simulink model "c172p"  (R2026a)
settings: configuration reference "standardSILConfiguraitonParams" (kept outside this file)
undefined symbols (not defined in the file): actuatorDelay_s, plantSampleTime_s
settings Model: Creator=GTAR  LastModifiedBy=Edison Altamirano
settings ConfigSetRef: SourceName=standardSILConfiguraitonParams  SourceLocation=Base Workspace

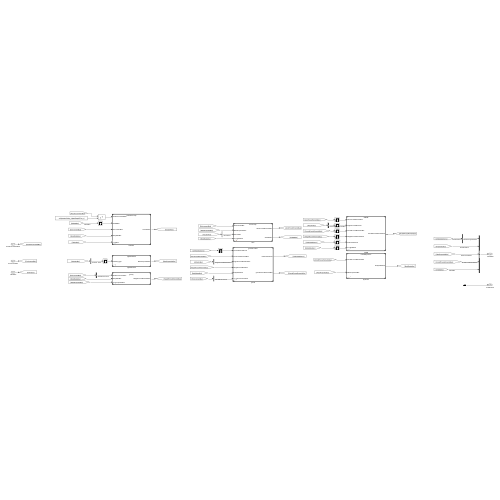
[thumbnail: Simulink's stored preview of the top-level diagram]
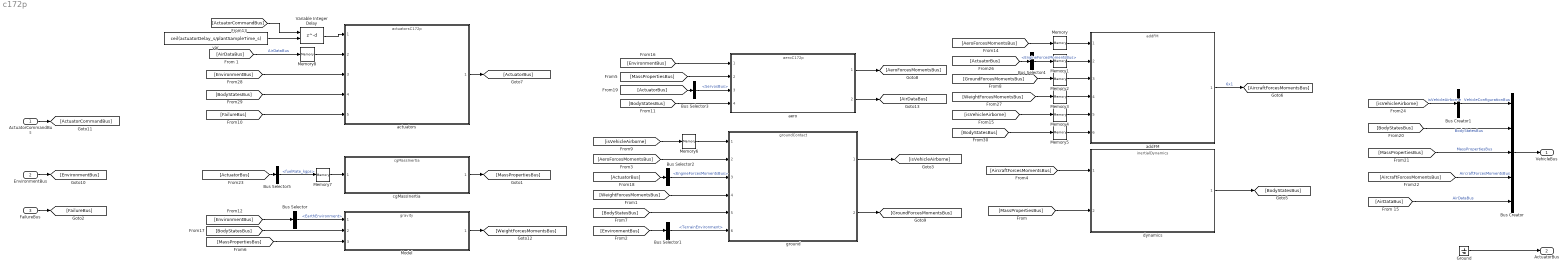
== system c172p ==
  ActuatorCommandBus : Inport  OutDataTypeStr=Bus: ActuatorCommandBus
  EnvironmentBus : Inport  Port=2  OutDataTypeStr=Bus: EnvironmentBus
  FailureBus : Inport  Port=3  OutDataTypeStr=Bus: FailureBus
  Bus Creator : BusCreator  Inputs=5  OutDataTypeStr=Bus: VehicleBus
  Bus Creator1 : BusCreator  Inputs=1  OutDataTypeStr=Bus: VehicleConfigurationBus
      settings: InheritFromInputs=off
  Bus Selector : BusSelector  OutputSignals=EarthEnvironment
  Bus Selector1 : BusSelector  OutputSignals=TerrainEnvironment
  Bus Selector2 : BusSelector  OutputSignals=PropulsionBus.EngineForcesMomentsBus
  Bus Selector3 : BusSelector  OutputSignals=ServosBus
  Bus Selector4 : BusSelector  OutputSignals=PropulsionBus.EngineForcesMomentsBus
  Bus Selector5 : BusSelector  OutputSignals=PropulsionBus.fuelRate_kgps
  Ground : Ground
  Memory{,1..8} (9 alike) : Memory
  Model : ModelReference  ModelNameDialog=gravity.slx  SimulationMode=Normal  ModelReferenceVersion=1.28
  Variable Integer Delay : Delay  DelayLengthSource=Input port
      settings: InputPortMap=u0,p1
  actuators : ModelReference  ModelNameDialog=actuatorsC172p.slx  SimulationMode=Normal  ModelReferenceVersion=5.0
  addFM : ModelReference  ModelNameDialog=addFM.slx  SimulationMode=Normal  ModelReferenceVersion=1.82
  aero : ModelReference  ModelNameDialog=aeroC172p.slx  SimulationMode=Normal  ModelReferenceVersion=5.0
  cgMassInertia : ModelReference  ModelNameDialog=cgMassInertia.slx  SimulationMode=Normal  ModelReferenceVersion=1.43
  dynamics : ModelReference  ModelNameDialog=inertialDynamics.slx  SimulationMode=Normal  ModelReferenceVersion=1.35
  ground : ModelReference  ModelNameDialog=groundContact.slx  SimulationMode=Normal  ModelReferenceVersion=1.99
  var : Constant  Value=ceil(actuatorDelay_s/plantSampleTime_s)
  VehicleBus : Outport  OutDataTypeStr=Bus: VehicleBus
  ActuatorBus : Outport  Port=2  OutDataTypeStr=Bus: ActuatorBus
  wires:
  actuators/1 -> [ActuatorBus]
  var/1 -> Variable Integer Delay/2
  Bus Selector3/1 -> aero/3  "<ServosBus>"
  [MassPropertiesBus] -> dynamics/2
  [MassPropertiesBus] -> aero/2
  Bus Creator/1 -> VehicleBus/1
  Variable Integer Delay/1 -> actuators/1
  addFM/1 -> [AircraftForcesMomentsBus]  "6x1"
  aero/1 -> [AeroForcesMomentsBus]
  [BodyStatesBus] -> aero/4
  EnvironmentBus/1 -> [EnvironmentBus]
  ActuatorCommandBus/1 -> [ActuatorCommandBus]
  [ActuatorCommandBus] -> Variable Integer Delay/1
  [AeroForcesMomentsBus] -> Memory/1
  [EnvironmentBus] -> aero/1
  Model/1 -> [WeightForcesMomentsBus]
  Bus Selector4/1 -> Memory1/1  "<EngineForcesMomentsBus>"
  [GroundForcesMomentsBus] -> Memory2/1
  ground/2 -> [GroundForcesMomentsBus]
  cgMassInertia/1 -> [MassPropertiesBus]
  ground/1 -> [isVehicleAirborne]
  Memory6/1 -> ground/1
  [isVehicleAirborne] -> Memory6/1
  [MassPropertiesBus] -> Model/3
  [EnvironmentBus] -> Bus Selector/1
  Bus Selector/1 -> Model/1  "<EarthEnvironment>"
  [BodyStatesBus] -> Model/2
  [EnvironmentBus] -> Bus Selector1/1
  [ActuatorBus] -> Bus Selector2/1
  [ActuatorBus] -> Bus Selector3/1
  [BodyStatesBus] -> Bus Creator/2  "BodyStatesBus"
  [MassPropertiesBus] -> Bus Creator/3  "MassPropertiesBus"
  [AircraftForcesMomentsBus] -> Bus Creator/4  "AircraftForcesMomentsBus"
  Bus Creator1/1 -> Bus Creator/1  "VehicleConfigurationBus"
  [isVehicleAirborne] -> Bus Creator1/1  "isVehicleAirborne"
  [ActuatorBus] -> Bus Selector4/1
  dynamics/1 -> [BodyStatesBus]
  aero/2 -> [AirDataBus]
  [AirDataBus] -> Bus Creator/5  "AirDataBus"
  [AircraftForcesMomentsBus] -> dynamics/1
  [ActuatorBus] -> Bus Selector5/1
  Bus Selector5/1 -> Memory7/1  "<fuelRate_kgps>"
  Memory7/1 -> cgMassInertia/1
  [WeightForcesMomentsBus] -> Memory3/1
  [AirDataBus] -> Memory8/1  "AirDataBus"
  [EnvironmentBus] -> actuators/3
  [BodyStatesBus] -> actuators/4
  Memory8/1 -> actuators/2
  [isVehicleAirborne] -> Memory4/1
  [BodyStatesBus] -> Memory5/1
  Ground/1 -> ActuatorBus/1
  [AeroForcesMomentsBus] -> ground/2
  Bus Selector2/1 -> ground/3  "<EngineForcesMomentsBus>"
  [WeightForcesMomentsBus] -> ground/4
  [BodyStatesBus] -> ground/5
  Bus Selector1/1 -> ground/6  "<TerrainEnvironment>"
  FailureBus/1 -> [FailureBus]
  [FailureBus] -> actuators/5
  Memory2/1 -> addFM/3
  Memory/1 -> addFM/1
  Memory1/1 -> addFM/2
  Memory3/1 -> addFM/4
  Memory4/1 -> addFM/5
  Memory5/1 -> addFM/6
